simulink model "chap6_2sim"  (Simulink 7.0)
settings: Solver=ode45  StartTime=0.0  StopTime=20  FixedStep=0.001  RelTol=1e-3
settings Model: Creator=Administrator  LastModifiedBy=eleliuj  ExtModeTrigMode=oneshot  ExtModeArmWhenConnect=off
settings DataIOCC: LimitDataPoints=off  SignalLoggingName=sigsOut
settings OptimizationCC: BooleanDataType=off
settings DebuggingCC: SaveWithParameterizedLinksMsg=none  SignalResolutionControl=TryResolveAllWithWarning  SolverPrmCheckMsg=none  MultiTaskDSMMsg=warning  MultiTaskCondExecSysMsg=none  StrictBusMsg=None
settings HardwareCC: TargetUnknown=on
settings RTWCC: IncludeERTFirstTime=on

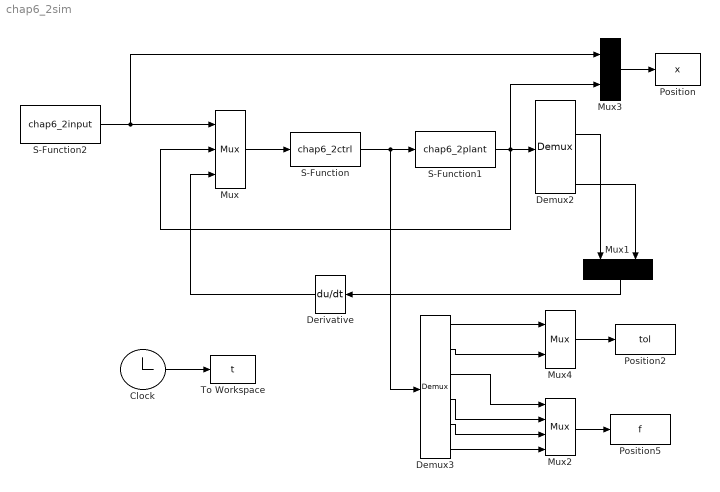
== system chap6_2sim ==
  Clock : Clock
      settings: Decimation=10
  Demux2 : Demux
  Demux3 : Demux  Outputs=6
  Derivative : Derivative  Orientation=left
  Mux : Mux  Inputs=3
  Mux1 : Mux  Orientation=down  Inputs=2
  Mux2 : Mux
  Mux3 : Mux  Inputs=2
  Mux4 : Mux  Inputs=2
  Position : ToWorkspace  VariableName=x  SampleTime=-1  SaveFormat=Array
  Position2 : ToWorkspace  VariableName=tol  SampleTime=-1  SaveFormat=Array
  Position5 : ToWorkspace  VariableName=f  SampleTime=-1  SaveFormat=Array
  S-Function : S-Function  FunctionName=chap6_2ctrl
  S-Function1 : S-Function  FunctionName=chap6_2plant
  S-Function2 : S-Function  FunctionName=chap6_2input
  To Workspace : ToWorkspace  VariableName=t  SampleTime=-1  SaveFormat=Array
  wires:
  Mux/1 -> S-Function/1
  Mux3/1 -> Position/1
  S-Function/1 -> S-Function1/1, Demux3/1
  S-Function1/1 -> Demux2/1, Mux3/2, Mux/2
  S-Function2/1 -> Mux3/1, Mux/1
  Demux2/2 -> Mux1/1
  Demux2/4 -> Mux1/2
  Mux1/1 -> Derivative/1
  Derivative/1 -> Mux/3
  Clock/1 -> To Workspace/1
  Mux2/1 -> Position5/1
  Demux3/3 -> Mux2/1
  Demux3/4 -> Mux2/2
  Demux3/5 -> Mux2/3
  Demux3/6 -> Mux2/4
  Mux4/1 -> Position2/1
  Demux3/1 -> Mux4/1
  Demux3/2 -> Mux4/2
